simulink model "Prova"  (R2019b)
settings: Solver=FixedStepAuto  StartTime=t(1)  StopTime=t(end)  FixedStep=0.005  RelTol=1e-3
model workspace (MAT data in the model file):
  tp10e9c9ed_669f_409e_ba1a_933f3c54d01d.time = 51799.88
  tp10e9c9ed_669f_409e_ba1a_933f3c54d01d.signals(1).values = 0
  tp10e9c9ed_669f_409e_ba1a_933f3c54d01d.signals(1).dimensions = 1
  tp10e9c9ed_669f_409e_ba1a_933f3c54d01d.signals(1).label = 'CSTATE'
  tp10e9c9ed_669f_409e_ba1a_933f3c54d01d.signals(1).blockName = 'Prova/Coulomb Counting/Integrator'
  tp10e9c9ed_669f_409e_ba1a_933f3c54d01d.signals(1).stateName = ''
  tp10e9c9ed_669f_409e_ba1a_933f3c54d01d.signals(1).inReferencedModel = 0
  tp10e9c9ed_669f_409e_ba1a_933f3c54d01d.signals(1).sampleTime = [0 0]
  tp10e9c9ed_669f_409e_ba1a_933f3c54d01d.signals(2).values = 0
  tp10e9c9ed_669f_409e_ba1a_933f3c54d01d.signals(2).dimensions = 1
  tp10e9c9ed_669f_409e_ba1a_933f3c54d01d.signals(2).label = 'CSTATE'
  tp10e9c9ed_669f_409e_ba1a_933f3c54d01d.signals(2).blockName = 'Prova/Cell/C1'
  tp10e9c9ed_669f_409e_ba1a_933f3c54d01d.signals(2).stateName = 'Prova.Cell.C1.vc'
  tp10e9c9ed_669f_409e_ba1a_933f3c54d01d.signals(2).inReferencedModel = 0
  tp10e9c9ed_669f_409e_ba1a_933f3c54d01d.signals(2).sampleTime = [0 0]
  tp10e9c9ed_669f_409e_ba1a_933f3c54d01d.signals(3).values = 0
  tp10e9c9ed_669f_409e_ba1a_933f3c54d01d.signals(3).dimensions = 1
  tp10e9c9ed_669f_409e_ba1a_933f3c54d01d.signals(3).label = 'CSTATE'
  tp10e9c9ed_669f_409e_ba1a_933f3c54d01d.signals(3).blockName = 'Prova/Cell/C2'
  tp10e9c9ed_669f_409e_ba1a_933f3c54d01d.signals(3).stateName = 'Prova.Cell.C2.vc'
  tp10e9c9ed_669f_409e_ba1a_933f3c54d01d.signals(3).inReferencedModel = 0
  tp10e9c9ed_669f_409e_ba1a_933f3c54d01d.signals(3).sampleTime = [0 0]
  tp10e9c9ed_669f_409e_ba1a_933f3c54d01d.signals(4).values = 0.0163149663951
  tp10e9c9ed_669f_409e_ba1a_933f3c54d01d.signals(4).dimensions = 1
  tp10e9c9ed_669f_409e_ba1a_933f3c54d01d.signals(4).label = 'CSTATE'
  tp10e9c9ed_669f_409e_ba1a_933f3c54d01d.signals(4).blockName = 'Prova/Cell/C1'
  tp10e9c9ed_669f_409e_ba1a_933f3c54d01d.signals(4).stateName = 'Prova.Cell.C1.i'
  tp10e9c9ed_669f_409e_ba1a_933f3c54d01d.signals(4).inReferencedModel = 0
  tp10e9c9ed_669f_409e_ba1a_933f3c54d01d.signals(4).sampleTime = [0 0]
  tp10e9c9ed_669f_409e_ba1a_933f3c54d01d.signals(5).values = 0
  tp10e9c9ed_669f_409e_ba1a_933f3c54d01d.signals(5).dimensions = 1
  tp10e9c9ed_669f_409e_ba1a_933f3c54d01d.signals(5).label = 'CSTATE'
  tp10e9c9ed_669f_409e_ba1a_933f3c54d01d.signals(5).blockName = 'Prova/Cell/R0'
  tp10e9c9ed_669f_409e_ba1a_933f3c54d01d.signals(5).stateName = 'Prova.Cell.R0.v'
  tp10e9c9ed_669f_409e_ba1a_933f3c54d01d.signals(5).inReferencedModel = 0
  tp10e9c9ed_669f_409e_ba1a_933f3c54d01d.signals(5).sampleTime = [0 0]
  tp10e9c9ed_669f_409e_ba1a_933f3c54d01d.signals(6).values = 0.023437685662
  tp10e9c9ed_669f_409e_ba1a_933f3c54d01d.signals(6).dimensions = 1
  tp10e9c9ed_669f_409e_ba1a_933f3c54d01d.signals(6).label = 'CSTATE'
  tp10e9c9ed_669f_409e_ba1a_933f3c54d01d.signals(6).blockName = 'Prova/Cell/C2'
  tp10e9c9ed_669f_409e_ba1a_933f3c54d01d.signals(6).stateName = 'Prova.Cell.C2.i'
  tp10e9c9ed_669f_409e_ba1a_933f3c54d01d.signals(6).inReferencedModel = 0
  tp10e9c9ed_669f_409e_ba1a_933f3c54d01d.signals(6).sampleTime = [0 0]
  tp10e9c9ed_669f_409e_ba1a_933f3c54d01d.signals(7).values = [0 0]
  tp10e9c9ed_669f_409e_ba1a_933f3c54d01d.signals(7).dimensions = 2
  tp10e9c9ed_669f_409e_ba1a_933f3c54d01d.signals(7).label = 'Discrete'
  tp10e9c9ed_669f_409e_ba1a_933f3c54d01d.signals(7).blockName = 'Prova/Solver
    | Configuration/EVAL_KEY/INPUT_1_1_1'
  tp10e9c9ed_669f_409e_ba1a_933f3c54d01d.signals(7).stateName = ''
  tp10e9c9ed_669f_409e_ba1a_933f3c54d01d.signals(7).inReferencedModel = 0
  tp10e9c9ed_669f_409e_ba1a_933f3c54d01d.signals(7).sampleTime = {[0 0]; [0.05 0]}
  tp10e9c9ed_669f_409e_ba1a_933f3c54d01d.signals(8).values = [1 -3.426721]
  tp10e9c9ed_669f_409e_ba1a_933f3c54d01d.signals(8).dimensions = 2
  tp10e9c9ed_669f_409e_ba1a_933f3c54d01d.signals(8).label = 'Discrete'
  tp10e9c9ed_669f_409e_ba1a_933f3c54d01d.signals(8).blockName = 'Prova/Solver
    | Configuration/EVAL_KEY/INPUT_7_1_1'
  tp10e9c9ed_669f_409e_ba1a_933f3c54d01d.signals(8).stateName = ''
  tp10e9c9ed_669f_409e_ba1a_933f3c54d01d.signals(8).inReferencedModel = 0
  tp10e9c9ed_669f_409e_ba1a_933f3c54d01d.signals(8).sampleTime = {[0 0]; [0.005 0]}
  tp10e9c9ed_669f_409e_ba1a_933f3c54d01d.signals(9).values = [0 0]
  tp10e9c9ed_669f_409e_ba1a_933f3c54d01d.signals(9).dimensions = 2
  tp10e9c9ed_669f_409e_ba1a_933f3c54d01d.signals(9).label = 'Discrete'
  tp10e9c9ed_669f_409e_ba1a_933f3c54d01d.signals(9).blockName = 'Prova/Solver
    | Configuration/EVAL_KEY/INPUT_2_1_1'
  tp10e9c9ed_669f_409e_ba1a_933f3c54d01d.signals(9).stateName = ''
  tp10e9c9ed_669f_409e_ba1a_933f3c54d01d.signals(9).inReferencedModel = 0
  tp10e9c9ed_669f_409e_ba1a_933f3c54d01d.signals(9).sampleTime = [0 0]
  tp10e9c9ed_669f_409e_ba1a_933f3c54d01d.signals(10).values = [0 0]
  tp10e9c9ed_669f_409e_ba1a_933f3c54d01d.signals(10).dimensions = 2
  tp10e9c9ed_669f_409e_ba1a_933f3c54d01d.signals(10).label = 'Discrete'
  tp10e9c9ed_669f_409e_ba1a_933f3c54d01d.signals(10).blockName = 'Prova/Solver
    | Configuration/EVAL_KEY/INPUT_5_1_1'
  tp10e9c9ed_669f_409e_ba1a_933f3c54d01d.signals(10).stateName = ''
  tp10e9c9ed_669f_409e_ba1a_933f3c54d01d.signals(10).inReferencedModel = 0
  tp10e9c9ed_669f_409e_ba1a_933f3c54d01d.signals(10).sampleTime = {[0 0]; [0.05 0]}
  tp10e9c9ed_669f_409e_ba1a_933f3c54d01d.signals(11).values = [0 0]
  tp10e9c9ed_669f_409e_ba1a_933f3c54d01d.signals(11).dimensions = 2
  tp10e9c9ed_669f_409e_ba1a_933f3c54d01d.signals(11).label = 'Discrete'
  tp10e9c9ed_669f_409e_ba1a_933f3c54d01d.signals(11).blockName = 'Prova/Solver
    | Configuration/EVAL_KEY/INPUT_6_1_1'
  tp10e9c9ed_669f_409e_ba1a_933f3c54d01d.signals(11).stateName = ''
  tp10e9c9ed_669f_409e_ba1a_933f3c54d01d.signals(11).inReferencedModel = 0
  tp10e9c9ed_669f_409e_ba1a_933f3c54d01d.signals(11).sampleTime = {[0 0]; [0.05 0]}
  tp10e9c9ed_669f_409e_ba1a_933f3c54d01d.signals(12).values = [0 0]
  tp10e9c9ed_669f_409e_ba1a_933f3c54d01d.signals(12).dimensions = 2
  tp10e9c9ed_669f_409e_ba1a_933f3c54d01d.signals(12).label = 'Discrete'
  tp10e9c9ed_669f_409e_ba1a_933f3c54d01d.signals(12).blockName = 'Prova/Solver
    | Configuration/EVAL_KEY/INPUT_3_1_1'
  tp10e9c9ed_669f_409e_ba1a_933f3c54d01d.signals(12).stateName = ''
  tp10e9c9ed_669f_409e_ba1a_933f3c54d01d.signals(12).inReferencedModel = 0
  tp10e9c9ed_669f_409e_ba1a_933f3c54d01d.signals(12).sampleTime = {[0 0]; [0.05 0]}
  tp10e9c9ed_669f_409e_ba1a_933f3c54d01d.signals(13).values = [0 0]
  tp10e9c9ed_669f_409e_ba1a_933f3c54d01d.signals(13).dimensions = 2
  tp10e9c9ed_669f_409e_ba1a_933f3c54d01d.signals(13).label = 'Discrete'
  tp10e9c9ed_669f_409e_ba1a_933f3c54d01d.signals(13).blockName = 'Prova/Solver
    | Configuration/EVAL_KEY/INPUT_4_1_1'
  tp10e9c9ed_669f_409e_ba1a_933f3c54d01d.signals(13).stateName = ''
  tp10e9c9ed_669f_409e_ba1a_933f3c54d01d.signals(13).inReferencedModel = 0
  tp10e9c9ed_669f_409e_ba1a_933f3c54d01d.signals(13).sampleTime = {[0 0]; [0.05 0]}
  tpd9f37093_83c5_4610_9fb4_27540475f98f.time = 51790.79
  tpd9f37093_83c5_4610_9fb4_27540475f98f.signals(1).values = 0
  tpd9f37093_83c5_4610_9fb4_27540475f98f.signals(1).dimensions = 1
  tpd9f37093_83c5_4610_9fb4_27540475f98f.signals(1).label = 'CSTATE'
  tpd9f37093_83c5_4610_9fb4_27540475f98f.signals(1).blockName = 'Prova/Coulomb Counting/Integrator'
  tpd9f37093_83c5_4610_9fb4_27540475f98f.signals(1).stateName = ''
  tpd9f37093_83c5_4610_9fb4_27540475f98f.signals(1).inReferencedModel = 0
  tpd9f37093_83c5_4610_9fb4_27540475f98f.signals(1).sampleTime = [0 0]
  tpd9f37093_83c5_4610_9fb4_27540475f98f.signals(2).values = 0
  tpd9f37093_83c5_4610_9fb4_27540475f98f.signals(2).dimensions = 1
  tpd9f37093_83c5_4610_9fb4_27540475f98f.signals(2).label = 'CSTATE'
  tpd9f37093_83c5_4610_9fb4_27540475f98f.signals(2).blockName = 'Prova/Cell/C1'
  tpd9f37093_83c5_4610_9fb4_27540475f98f.signals(2).stateName = 'Prova.Cell.C1.vc'
  tpd9f37093_83c5_4610_9fb4_27540475f98f.signals(2).inReferencedModel = 0
  tpd9f37093_83c5_4610_9fb4_27540475f98f.signals(2).sampleTime = [0 0]
  tpd9f37093_83c5_4610_9fb4_27540475f98f.signals(3).values = 0
  tpd9f37093_83c5_4610_9fb4_27540475f98f.signals(3).dimensions = 1
  tpd9f37093_83c5_4610_9fb4_27540475f98f.signals(3).label = 'CSTATE'
  tpd9f37093_83c5_4610_9fb4_27540475f98f.signals(3).blockName = 'Prova/Cell/C2'
  tpd9f37093_83c5_4610_9fb4_27540475f98f.signals(3).stateName = 'Prova.Cell.C2.vc'
  tpd9f37093_83c5_4610_9fb4_27540475f98f.signals(3).inReferencedModel = 0
  tpd9f37093_83c5_4610_9fb4_27540475f98f.signals(3).sampleTime = [0 0]
  tpd9f37093_83c5_4610_9fb4_27540475f98f.signals(4).values = -0.0652398714737
  tpd9f37093_83c5_4610_9fb4_27540475f98f.signals(4).dimensions = 1
  tpd9f37093_83c5_4610_9fb4_27540475f98f.signals(4).label = 'CSTATE'
  tpd9f37093_83c5_4610_9fb4_27540475f98f.signals(4).blockName = 'Prova/Cell/C1'
  tpd9f37093_83c5_4610_9fb4_27540475f98f.signals(4).stateName = 'Prova.Cell.C1.i'
  tpd9f37093_83c5_4610_9fb4_27540475f98f.signals(4).inReferencedModel = 0
  tpd9f37093_83c5_4610_9fb4_27540475f98f.signals(4).sampleTime = [0 0]
  tpd9f37093_83c5_4610_9fb4_27540475f98f.signals(5).values = 0
  tpd9f37093_83c5_4610_9fb4_27540475f98f.signals(5).dimensions = 1
  tpd9f37093_83c5_4610_9fb4_27540475f98f.signals(5).label = 'CSTATE'
  tpd9f37093_83c5_4610_9fb4_27540475f98f.signals(5).blockName = 'Prova/Cell/R0'
  tpd9f37093_83c5_4610_9fb4_27540475f98f.signals(5).stateName = 'Prova.Cell.R0.v'
  tpd9f37093_83c5_4610_9fb4_27540475f98f.signals(5).inReferencedModel = 0
  tpd9f37093_83c5_4610_9fb4_27540475f98f.signals(5).sampleTime = [0 0]
  tpd9f37093_83c5_4610_9fb4_27540475f98f.signals(6).values = 0.0329742883686
  tpd9f37093_83c5_4610_9fb4_27540475f98f.signals(6).dimensions = 1
  tpd9f37093_83c5_4610_9fb4_27540475f98f.signals(6).label = 'CSTATE'
  tpd9f37093_83c5_4610_9fb4_27540475f98f.signals(6).blockName = 'Prova/Cell/C2'
  tpd9f37093_83c5_4610_9fb4_27540475f98f.signals(6).stateName = 'Prova.Cell.C2.i'
  tpd9f37093_83c5_4610_9fb4_27540475f98f.signals(6).inReferencedModel = 0
  tpd9f37093_83c5_4610_9fb4_27540475f98f.signals(6).sampleTime = [0 0]
  tpd9f37093_83c5_4610_9fb4_27540475f98f.signals(7).values = [0 0]
  tpd9f37093_83c5_4610_9fb4_27540475f98f.signals(7).dimensions = 2
  tpd9f37093_83c5_4610_9fb4_27540475f98f.signals(7).label = 'Discrete'
  tpd9f37093_83c5_4610_9fb4_27540475f98f.signals(7).blockName = 'Prova/Solver
    | Configuration/EVAL_KEY/INPUT_1_1_1'
  tpd9f37093_83c5_4610_9fb4_27540475f98f.signals(7).stateName = ''
  tpd9f37093_83c5_4610_9fb4_27540475f98f.signals(7).inReferencedModel = 0
  tpd9f37093_83c5_4610_9fb4_27540475f98f.signals(7).sampleTime = {[0 0]; [0.05 0]}
  tpd9f37093_83c5_4610_9fb4_27540475f98f.signals(8).values = [1 -3.115955]
  tpd9f37093_83c5_4610_9fb4_27540475f98f.signals(8).dimensions = 2
  tpd9f37093_83c5_4610_9fb4_27540475f98f.signals(8).label = 'Discrete'
  tpd9f37093_83c5_4610_9fb4_27540475f98f.signals(8).blockName = 'Prova/Solver
    | Configuration/EVAL_KEY/INPUT_7_1_1'
  tpd9f37093_83c5_4610_9fb4_27540475f98f.signals(8).stateName = ''
  tpd9f37093_83c5_4610_9fb4_27540475f98f.signals(8).inReferencedModel = 0
  tpd9f37093_83c5_4610_9fb4_27540475f98f.signals(8).sampleTime = {[0 0]; [0.005 0]}
  tpd9f37093_83c5_4610_9fb4_27540475f98f.signals(9).values = [0 0]
  tpd9f37093_83c5_4610_9fb4_27540475f98f.signals(9).dimensions = 2
  tpd9f37093_83c5_4610_9fb4_27540475f98f.signals(9).label = 'Discrete'
  tpd9f37093_83c5_4610_9fb4_27540475f98f.signals(9).blockName = 'Prova/Solver
    | Configuration/EVAL_KEY/INPUT_2_1_1'
  tpd9f37093_83c5_4610_9fb4_27540475f98f.signals(9).stateName = ''
  tpd9f37093_83c5_4610_9fb4_27540475f98f.signals(9).inReferencedModel = 0
  tpd9f37093_83c5_4610_9fb4_27540475f98f.signals(9).sampleTime = {[0 0]; [0.05 0]}
  tpd9f37093_83c5_4610_9fb4_27540475f98f.signals(10).values = [0 0]
  tpd9f37093_83c5_4610_9fb4_27540475f98f.signals(10).dimensions = 2
  tpd9f37093_83c5_4610_9fb4_27540475f98f.signals(10).label = 'Discrete'
  tpd9f37093_83c5_4610_9fb4_27540475f98f.signals(10).blockName = 'Prova/Solver
    | Configuration/EVAL_KEY/INPUT_5_1_1'
  tpd9f37093_83c5_4610_9fb4_27540475f98f.signals(10).stateName = ''
  tpd9f37093_83c5_4610_9fb4_27540475f98f.signals(10).inReferencedModel = 0
  tpd9f37093_83c5_4610_9fb4_27540475f98f.signals(10).sampleTime = {[0 0]; [0.05 0]}
  tpd9f37093_83c5_4610_9fb4_27540475f98f.signals(11).values = [0 0]
  tpd9f37093_83c5_4610_9fb4_27540475f98f.signals(11).dimensions = 2
  tpd9f37093_83c5_4610_9fb4_27540475f98f.signals(11).label = 'Discrete'
  tpd9f37093_83c5_4610_9fb4_27540475f98f.signals(11).blockName = 'Prova/Solver
    | Configuration/EVAL_KEY/INPUT_6_1_1'
  tpd9f37093_83c5_4610_9fb4_27540475f98f.signals(11).stateName = ''
  tpd9f37093_83c5_4610_9fb4_27540475f98f.signals(11).inReferencedModel = 0
  tpd9f37093_83c5_4610_9fb4_27540475f98f.signals(11).sampleTime = {[0 0]; [0.05 0]}
  tpd9f37093_83c5_4610_9fb4_27540475f98f.signals(12).values = [0 0]
  tpd9f37093_83c5_4610_9fb4_27540475f98f.signals(12).dimensions = 2
  tpd9f37093_83c5_4610_9fb4_27540475f98f.signals(12).label = 'Discrete'
  tpd9f37093_83c5_4610_9fb4_27540475f98f.signals(12).blockName = 'Prova/Solver
    | Configuration/EVAL_KEY/INPUT_3_1_1'
  tpd9f37093_83c5_4610_9fb4_27540475f98f.signals(12).stateName = ''
  tpd9f37093_83c5_4610_9fb4_27540475f98f.signals(12).inReferencedModel = 0
  tpd9f37093_83c5_4610_9fb4_27540475f98f.signals(12).sampleTime = {[0 0]; [0.05 0]}
  tpd9f37093_83c5_4610_9fb4_27540475f98f.signals(13).values = [0 0]
  tpd9f37093_83c5_4610_9fb4_27540475f98f.signals(13).dimensions = 2
  tpd9f37093_83c5_4610_9fb4_27540475f98f.signals(13).label = 'Discrete'
  tpd9f37093_83c5_4610_9fb4_27540475f98f.signals(13).blockName = 'Prova/Solver
    | Configuration/EVAL_KEY/INPUT_4_1_1'
  tpd9f37093_83c5_4610_9fb4_27540475f98f.signals(13).stateName = ''
  tpd9f37093_83c5_4610_9fb4_27540475f98f.signals(13).inReferencedModel = 0
  tpd9f37093_83c5_4610_9fb4_27540475f98f.signals(13).sampleTime = {[0 0]; [0.05 0]}
values from neighbouring files (symbols this model uses):
  C1_lut = [2616.79512849 2616.43283088 2615.59967331 2614.47435321 2613.3431375 2612.62601033 2612.96267669 2615.42855098 2622.05730089 2637.46024935 2673.00916395 2819.35300715 ... (4000 elements, 100x40)]    [New_LUT.mat]    (also in New_LUT_2_better.mat)
  C2_lut = [8316.55282172 8241.37270216 8044.69907261 7701.04533683 7155.44227693 6280.64344837 4764.65772311 150.204385688 4996.010408 6768.13209087 7991.23230792 10485.0523663 ... (4000 elements, 100x40)]    [New_LUT.mat]    (also in New_LUT_2_better.mat)
  OCV_lut = [2.54020422692 2.68040845384 2.81538392295 2.88895607028 2.94916911681 2.99822851777 3.0372449808 3.07029327569 3.09992793679 3.12541619029 3.15027805329 3.1746347997 ... (100 elements, 100x1)]    [New_LUT.mat]    (also in New_LUT_2_better.mat)
  R0_est = 0    [PEst_2.m]
  R1_lut = [0.00288289613177 0.00288389755685 0.00288641797479 0.00289050028449 0.00289621540381 0.00290366565505 0.00291298991178 0.00292437107831 0.00293804680593 0.00295432488141 0.00297360560985 0.00299641505789 ... (4000 elements, 100x40)]    [New_LUT.mat]    (also in New_LUT_2_better.mat = [0.0288289613177 0.0288389755685 0.0288641797479 0.028905002)
  R2_lut = [0.00245662570125 0.00245712328256 0.00245838533692 0.00246045866117 0.00246342298728 0.00246739904613 0.00247256292524 0.00247917203717 0.00248761479657 0.00249851493602 0.00251297509684 0.00253333733005 ... (4000 elements, 100x40)]    [New_LUT.mat]    (also in New_LUT_2_better.mat = [0.0245662570125 0.0245712328256 0.0245838533692 0.024604586)
  SOC_lut = [0 2.91262135922 3.21380154603 3.51498173285 3.831220929 4.26793219987 4.68205495674 4.98323514355 5.39735790041 5.84912818063 6.37619350755 6.97855388117 ... (117 elements, 117x1)]    [New_LUT.mat]    (also in New_LUT_2_better.mat)
  v = Voltage((i+p):(step+p))    [PEst_2.m]
undefined symbols (not defined in the file or in its folder): Est
libraries: nesl_utility x14, fl_lib x12, ee_lib x2
settings Model: OrderedModelArguments=off  Creator=Utente  LastModifiedBy=PcElettronicaDynamis
settings DataIOCC: InitialState=tpd9f37093_83c5_4610_9fb4_27540475f98f  LoadInitialState=on  SaveOutput=off  DSMLogging=off  InspectSignalLogs=on  OutputOption=AdditionalOutputTimes  OutputTimes=SDO_OutputTimes  ReturnWorkspaceOutputsName=SDOSimTest_Log

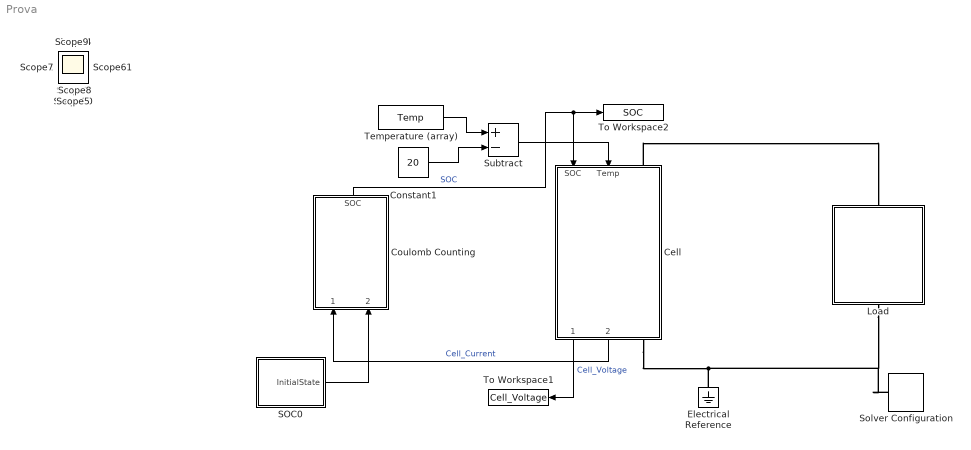
== system Prova ==
  Cell : Subsystem
  Constant1 : Constant  Value=20  SampleTime=0.005
  Coulomb Counting : Subsystem
  Electrical Reference : fl_lib/Electrical/Electrical Elements/Electrical Reference
  Load : Subsystem
  SOC0 : Subsystem
  Solver Configuration : nesl_utility/Solver Configuration  PhysicalDomain=network_engine_domain  SubClassName=solver  LeftPortType=input  RightPortType=generic  Tones=[]  Harmonics=[]  SimulateNoise=off  Profile=off  UseLocalSampling=off  EnableSwitchedLinearOptims=on  FrequencyDomain=off  UseCCode=off  RelTol=0.001  AbsTol=1e-06  MinStep=1e-09  ToWorkspace=off  RevertToSquareIcSolve=off  NumHomotopyIterations=100  PhasorMode=off  PhasorModeNumHarmonics=1  DoDC=off  ResidualTolerance=1e-09  UseLocalSolver=off  LocalSolverChoice=NE_BACKWARD_EULER_ADVANCER  LocalSolverSampleTime=0.001  DoFixedCost=off  MaxNonlinIter=3  MaxModeIter=2  LinearAlgebra=auto  EquationFormulation=NE_TIME_EF  DelaysMemoryBudget=1024  AutomaticFiltering=on  FilteringTimeConstant=0.001  PartitionStorageMethod=AS_NEEDED  PartitionMemoryBudget=1024  PartitionMethod=ROBUST
  Subtract : Sum  Inputs=+-
  Temperature (array) : FromWorkspace  VariableName=Temp  SampleTime=0.005
  To Workspace1 : ToWorkspace  VariableName=Cell_Voltage  SaveFormat=Timeseries  SampleTime=0.005
  To Workspace2 : ToWorkspace  VariableName=SOC  SaveFormat=Timeseries  SampleTime=0.005
  Scope{,1..11} (12 alike) : Scope
  wires:
  Cell/2(Cell_Current) -> Coulomb Counting/1(Cell_Current)  "Cell_Current"
  Coulomb Counting/1(SOC) -> To Workspace2/1, Cell/1(SOC)  "SOC"
  Cell/1(Cell_Voltage) -> To Workspace1/1  "Cell_Voltage"
  SOC0/1(InitialState) -> Coulomb Counting/2(InitialState)
  Temperature (array)/1 -> Subtract/1
  Constant1/1 -> Subtract/2
  Subtract/1 -> Cell/2(Temp)
  connections:
  Electrical Reference/LConn1 -- Cell/RConn1 -- Solver Configuration/RConn1 -- Load/LConn1
  Cell/LConn1 -- Load/RConn1

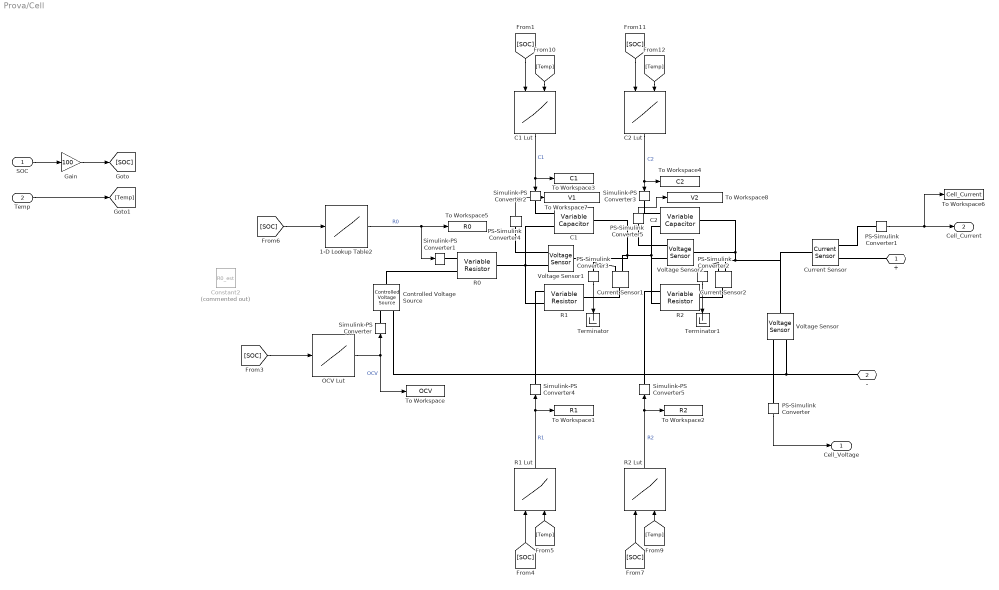
== system Prova/Cell ==
  SOC : Inport  SampleTime=0.05
  Temp : Inport  Port=2  SampleTime=0.05
  1-D Lookup Table2 : Lookup_n-D  NumberOfTableDimensions=1  BreakpointsForDimension1=[1:1800:57600]  Table=Est(:,1)  InternalRulePriority=Speed  RndMeth=Simplest  InputSameDT=on
  C1 : ee_lib/Passive/Variable Capacitor  prm=2  Cmin=1e-9 F  r=1e-6 Ohm  v0=0 V  q0=0 C
      settings: SourceProductName=Simscape Electrical  SourceProductBaseCode=PS  InternalSimscapePortConfiguration="{\"Bottom\":[],\"Left\":[{\"id\":\"C\",\"label\":\"C\",\"type\":\"input\"},{\"id\":\"p\",\"label\":\"+\",\"type\":\"foundation.electrical.electrical\"}],\"Right\":[{\"id\":\"n\",\"label\":\"-\",\"type\":\"foundation.electrical.electrical\"}],\"Top\":[]}"
  C1 Lut : Lookup_n-D  BreakpointsForDimension1=[1:100]  BreakpointsForDimension2=[1:40]  Table=C1_lut  RndMeth=Simplest  InputSameDT=on
  C2 : ee_lib/Passive/Variable Capacitor  prm=2  Cmin=1e-9 F  r=1e-6 Ohm  v0=0 V  q0=0 C
      settings: SourceProductName=Simscape Electrical  SourceProductBaseCode=PS  InternalSimscapePortConfiguration="{\"Bottom\":[],\"Left\":[{\"id\":\"C\",\"label\":\"C\",\"type\":\"input\"},{\"id\":\"p\",\"label\":\"+\",\"type\":\"foundation.electrical.electrical\"}],\"Right\":[{\"id\":\"n\",\"label\":\"-\",\"type\":\"foundation.electrical.electrical\"}],\"Top\":[]}"
  C2 Lut : Lookup_n-D  BreakpointsForDimension1=[1:100]  BreakpointsForDimension2=[1:40]  Table=C2_lut  RndMeth=Simplest  InputSameDT=on
  Constant2 : Constant  Commented=on  Value=R0_est
  Controlled Voltage Source : fl_lib/Electrical/Electrical Sources/Controlled Voltage Source
  Current Sensor : fl_lib/Electrical/Electrical Sensors/Current Sensor
  Current Sensor1 : fl_lib/Electrical/Electrical Sensors/Current Sensor
  Current Sensor2 : fl_lib/Electrical/Electrical Sensors/Current Sensor
  Gain : Gain  Gain=100
  OCV Lut : Lookup_n-D  NumberOfTableDimensions=1  BreakpointsForDimension1=[1:100]  Table=OCV_lut  InternalRulePriority=Speed  RndMeth=Simplest  InputSameDT=on
  PS-Simulink Converter{,1..5} (6 alike) : nesl_utility/PS-Simulink Converter  PhysicalDomain=network_engine_domain  SubClassName=ps_output  LeftPortType=input  RightPortType=output  PseudoPeriodic=off  Frequencies=[]  Unit=inherit  AffineConversion=off
  R0 : fl_lib/Electrical/Electrical Elements/Variable Resistor  Rmin=0 Ohm  i_specify=off  i_priority=None  i=0 A  i_nominal_specify=off  i_nominal_unit=A  i_nominal_value=1  v_specify=off  v_priority=None  v=0 V  v_nominal_specify=off  v_nominal_unit=V  v_nominal_value=1
  R1 : fl_lib/Electrical/Electrical Elements/Variable Resistor  Rmin=0 Ohm  i_specify=off  i_priority=None  i=0 A  i_nominal_specify=off  i_nominal_unit=A  i_nominal_value=1  v_specify=off  v_priority=None  v=0 V  v_nominal_specify=off  v_nominal_unit=V  v_nominal_value=1
  R1 Lut : Lookup_n-D  BreakpointsForDimension1=[1:100]  BreakpointsForDimension2=[1:40]  Table=R1_lut  RndMeth=Simplest  InputSameDT=on
  R2 : fl_lib/Electrical/Electrical Elements/Variable Resistor  Rmin=0 Ohm  i_specify=off  i_priority=None  i=0 A  i_nominal_specify=off  i_nominal_unit=A  i_nominal_value=1  v_specify=off  v_priority=None  v=0 V  v_nominal_specify=off  v_nominal_unit=V  v_nominal_value=1
  R2 Lut : Lookup_n-D  BreakpointsForDimension1=[1:100]  BreakpointsForDimension2=[1:40]  Table=R2_lut  RndMeth=Simplest  InputSameDT=on
  Simulink-PS Converter{,1..5} (6 alike) : nesl_utility/Simulink-PS Converter  PhysicalDomain=network_engine_domain  SubClassName=ps_input  LeftPortType=input  RightPortType=output  PseudoPeriodic=off  Frequencies=[]  NoiseDistribution=none  NoiseParameters=[]  Unit=1  AffineConversion=off  FilteringAndDerivatives=provide  SimscapeFilterOrder=1  InputFilterTimeConstant=0.001  UdotUserProvided=0
  Terminator : Terminator
  Terminator1 : Terminator
  To Workspace : ToWorkspace  VariableName=OCV  SaveFormat=Timeseries  SampleTime=0.005
  To Workspace1 : ToWorkspace  VariableName=R1  SaveFormat=Timeseries  SampleTime=0.005
  To Workspace2 : ToWorkspace  VariableName=R2  SaveFormat=Timeseries  SampleTime=0.005
      settings: MaxDataPoints=Inf
  To Workspace3 : ToWorkspace  VariableName=C1  SaveFormat=Timeseries  SampleTime=0.005
  To Workspace4 : ToWorkspace  VariableName=C2  SaveFormat=Timeseries  SampleTime=0.005
  To Workspace5 : ToWorkspace  VariableName=R0  SaveFormat=Timeseries  SampleTime=0.005
  To Workspace6 : ToWorkspace  VariableName=Cell_Current  SaveFormat=Timeseries  SampleTime=0.005
  To Workspace7 : ToWorkspace  VariableName=V1  SaveFormat=Timeseries  SampleTime=-1
  To Workspace8 : ToWorkspace  VariableName=V2  SaveFormat=Timeseries  SampleTime=-1
  Voltage Sensor : fl_lib/Electrical/Electrical Sensors/Voltage Sensor
  Voltage Sensor1 : fl_lib/Electrical/Electrical Sensors/Voltage Sensor
  Voltage Sensor2 : fl_lib/Electrical/Electrical Sensors/Voltage Sensor
  + : PMIOPort  Side=Left
  - : PMIOPort  Port=2  Side=Right
  Cell_Voltage : Outport  SampleTime=0.05
  Cell_Current : Outport  Port=2  SampleTime=0.05
  wires:
  PS-Simulink Converter/1 -> Cell_Voltage/1
  R1 Lut/1 -> To Workspace1/1, Simulink-PS Converter4/1  "R1"
  OCV Lut/1 -> To Workspace/1, Simulink-PS Converter/1  "OCV"
  1-D Lookup Table2/1 -> To Workspace5/1, Simulink-PS Converter1/1  "R0"
  R2 Lut/1 -> Simulink-PS Converter5/1, To Workspace2/1  "R2"
  PS-Simulink Converter1/1 -> To Workspace6/1, Cell_Current/1
  Gain/1 -> [SOC]
  C2 Lut/1 -> To Workspace4/1, Simulink-PS Converter3/1  "C2"
  C1 Lut/1 -> Simulink-PS Converter2/1, To Workspace3/1  "C1"
  [SOC] -> OCV Lut/1
  SOC/1 -> Gain/1
  PS-Simulink Converter3/1 -> Terminator/1
  PS-Simulink Converter2/1 -> Terminator1/1
  [SOC] -> C2 Lut/1
  [SOC] -> C1 Lut/1
  [Temp] -> C1 Lut/2
  [Temp] -> C2 Lut/2
  [SOC] -> R2 Lut/1
  [SOC] -> R1 Lut/1
  [Temp] -> R1 Lut/2
  Temp/1 -> [Temp]
  [Temp] -> R2 Lut/2
  PS-Simulink Converter4/1 -> To Workspace7/1
  PS-Simulink Converter5/1 -> To Workspace8/1
  [SOC] -> 1-D Lookup Table2/1
  connections:
  C1/RConn1 -- Voltage Sensor2/RConn2 -- R2/LConn2 -- C2/LConn2 -- Voltage Sensor1/LConn1 -- Current Sensor1/RConn2
  Current Sensor/LConn1 -- Voltage Sensor/LConn1 -- Current Sensor2/RConn2 -- Voltage Sensor2/LConn1 -- C2/RConn1
  R0/RConn1 -- C1/LConn2 -- Voltage Sensor1/RConn2 -- R1/LConn2
  Simulink-PS Converter3/RConn1 -- C2/LConn1
  Controlled Voltage Source/RConn2 -- Voltage Sensor/RConn2 -- -/RConn1
  Simulink-PS Converter5/RConn1 -- R2/LConn1
  PS-Simulink Converter/LConn1 -- Voltage Sensor/RConn1
  Simulink-PS Converter2/RConn1 -- C1/LConn1
  Simulink-PS Converter1/RConn1 -- R0/LConn1
  R1/LConn1 -- Simulink-PS Converter4/RConn1
  Simulink-PS Converter/RConn1 -- Controlled Voltage Source/RConn1
  Controlled Voltage Source/LConn1 -- R0/LConn2
  PS-Simulink Converter1/LConn1 -- Current Sensor/RConn1
  Current Sensor/RConn2 -- +/RConn1
  Current Sensor1/LConn1 -- R1/RConn1
  Current Sensor2/LConn1 -- R2/RConn1
  Current Sensor2/RConn1 -- PS-Simulink Converter2/LConn1
  PS-Simulink Converter3/LConn1 -- Current Sensor1/RConn1
  PS-Simulink Converter4/LConn1 -- Voltage Sensor1/RConn1
  PS-Simulink Converter5/LConn1 -- Voltage Sensor2/RConn1

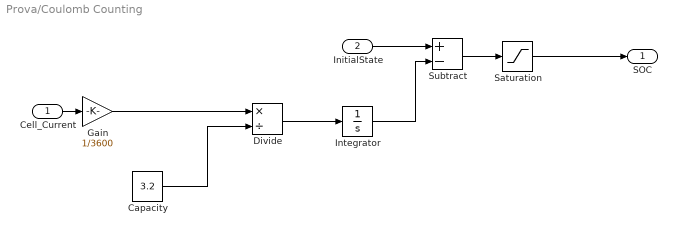
== system Prova/Coulomb Counting ==
  Cell_Current : Inport  SampleTime=0.05
  InitialState : Inport  Port=2
  Capacity : Constant  Value=3.2
  Divide : Product  Inputs=*/
  Gain : Gain  Gain=1/3600
  Integrator : Integrator
  Saturation : Saturate  UpperLimit=1  LowerLimit=0
  Subtract : Sum  Inputs=+-
  SOC : Outport  SampleTime=0.05  VectorParamsAs1DForOutWhenUnconnected=off
  wires:
  Divide/1 -> Integrator/1
  Cell_Current/1 -> Gain/1
  Subtract/1 -> Saturation/1
  Integrator/1 -> Subtract/2
  Capacity/1 -> Divide/2
  InitialState/1 -> Subtract/1
  Saturation/1 -> SOC/1
  Gain/1 -> Divide/1

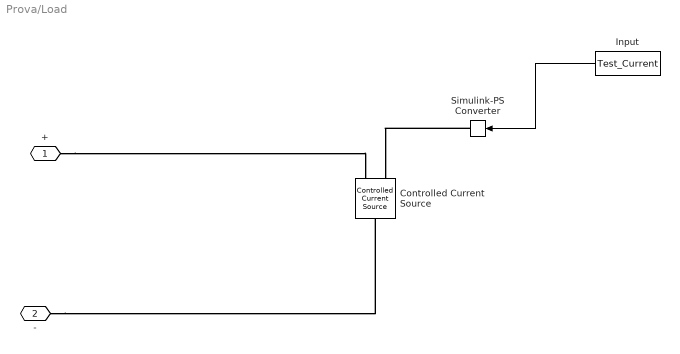
== system Prova/Load ==
  Controlled Current Source : fl_lib/Electrical/Electrical Sources/Controlled Current Source
  Input : FromWorkspace  VariableName=Test_Current  SampleTime=0.005
  Simulink-PS Converter : nesl_utility/Simulink-PS Converter  PhysicalDomain=network_engine_domain  SubClassName=ps_input  LeftPortType=input  RightPortType=output  PseudoPeriodic=off  Frequencies=[]  NoiseDistribution=none  NoiseParameters=[]  Unit=1  AffineConversion=off  FilteringAndDerivatives=provide  SimscapeFilterOrder=1  InputFilterTimeConstant=0.001  UdotUserProvided=0
  + : PMIOPort  Side=Right
  - : PMIOPort  Port=2  Side=Left
  wires:
  Input/1 -> Simulink-PS Converter/1
  connections:
  +/RConn1 -- Controlled Current Source/RConn2
  Simulink-PS Converter/RConn1 -- Controlled Current Source/RConn1
  -/RConn1 -- Controlled Current Source/LConn1

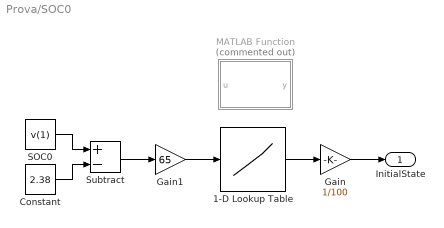
== system Prova/SOC0 ==
  1-D Lookup Table : Lookup_n-D  NumberOfTableDimensions=1  BreakpointsForDimension1=[1:117]  Table=SOC_lut  InternalRulePriority=Speed  RndMeth=Simplest  InputSameDT=on
  Constant : Constant  Value=2.38  SampleTime=0.005
  Gain : Gain  Gain=1/100
  Gain1 : Gain  Gain=65
  MATLAB Function : MATLAB Function  Commented=on  TreatAsAtomicUnit=on
  SOC0 : Constant  Value=v(1)  SampleTime=0.005
  Subtract : Sum  Inputs=+-
  InitialState : Outport
  wires:
  1-D Lookup Table/1 -> Gain/1
  Gain/1 -> InitialState/1
  Gain1/1 -> 1-D Lookup Table/1
  Subtract/1 -> Gain1/1
  SOC0/1 -> Subtract/1
  Constant/1 -> Subtract/2

== matlab function Prova/SOC0/MATLAB Function ==
  data: u input; y output
function y = setState(u)
y = 0;
y(1,1) = interp1(sococv(1:117,2), sococv(1:117,1), u);

end
